simulink model "test"  (R2019b)
settings: Solver=VariableStepAuto  StartTime=0.0  StopTime=0.05  RelTol=1e-3
libraries: powerlib x11, simulink x3, dspsigops x1
settings Model: Creator=29721  LastModifiedBy=29721

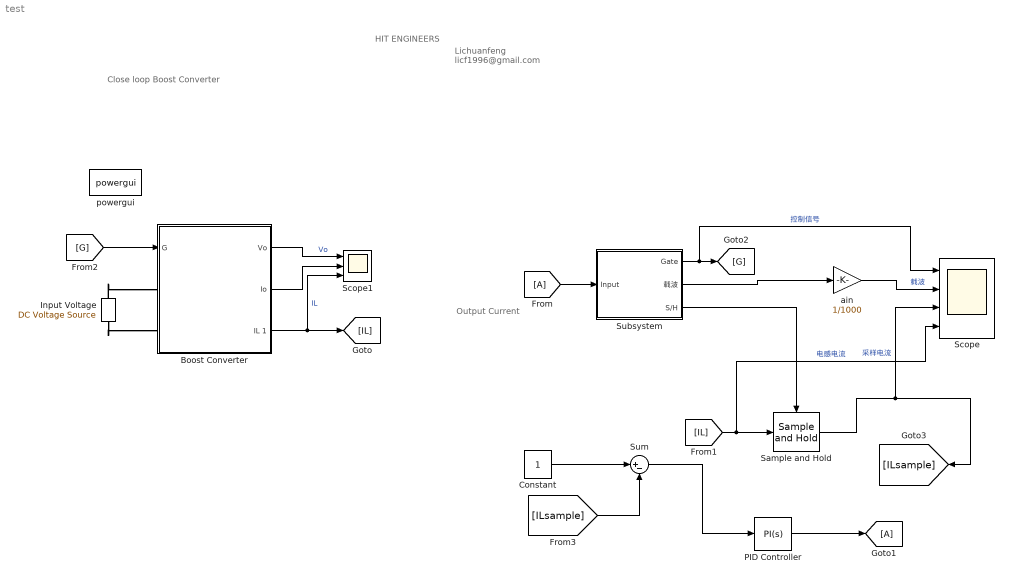
== system test ==
  note: HIT
      | ENGINEERS
  note: Lichuanfeng
      | licf1996@gmail.com
  note: Output Current
  note: Close loop Boost Converter
  Boost Converter : Subsystem  mask{R=20, L=5000e-6, C=220e-6}
      mask prompts: R "Resitor"; L "Inductor"; C "Capacitor"
  Constant : Constant
  Input Voltage : powerlib/Electrical Sources/DC Voltage Source  Amplitude=5  Measurements=None
  PID Controller : simulink/Continuous/PID Controller  Controller=PI  Form=Parallel  TimeDomain=Continuous-time  SampleTime=-1  IntegratorMethod=Forward Euler  FilterMethod=Forward Euler  ControllerParametersSource=internal  P=5000  I=20000  D=0  UseFilter=on  N=100  TunerSelectOption=Transfer Function Based (PID Tuner App)  InitialConditionSource=internal  InitialConditionForIntegrator=0  InitialConditionForFilter=0  DifferentiatorICPrevScaledInput=0  ExternalReset=none  TrackingMode=off  Kt=1  LimitOutput=off  UpperSaturationLimit=inf  LowerSaturationLimit=-inf  LinearizeAsGain=on  AntiWindupMode=none  Kb=1  POutMin=[]  POutMax=[]  IOutMin=[]  IOutMax=[]  DOutMin=[]  DOutMax=[]  NOutMin=[]  NOutMax=[]  SumOutMin=[]  SumOutMax=[]  SaturationOutMin=[]  SaturationOutMax=[]  PParamMin=[]  PParamMax=[]  IParamMin=[]  IParamMax=[]  DParamMin=[]  DParamMax=[]  NParamMin=[]  NParamMax=[]  KbParamMin=[]  KbParamMax=[]  KtParamMin=[]  KtParamMax=[]  KbOutMin=[]  KbOutMax=[]  KtOutMin=[]  KtOutMax=[]  IntegratorOutMin=[]  IntegratorOutMax=[]  FilterOutMin=[]  FilterOutMax=[]  SumI1OutMin=[]  SumI1OutMax=[]  SumI2OutMin=[]  SumI2OutMax=[]  SumI3OutMin=[]  SumI3OutMax=[]  SumI4OutMin=[]  SumI4OutMax=[]  SumDOutMin=[]  SumDOutMax=[]  DifferentiatorOutMin=[]  DifferentiatorOutMax=[]  FilterDiffOutCoefMin=[]  FilterDiffOutCoefMax=[]  ReciprocalOutMin=[]  ReciprocalOutMax=[]  SumDenOutMin=[]  SumDenOutMax=[]  SumNumOutMin=[]  SumNumOutMax=[]  DivideOutMin=[]  DivideOutMax=[]  IntegratorContinuousStateAttributes=''  IntegratorStateMustResolveToSignalObject=off  IntegratorRTWStateStorageClass=Auto  FilterContinuousStateAttributes=''  FilterStateMustResolveToSignalObject=off  FilterRTWStateStorageClass=Auto  ParallelPVariant=InternalParameters  IdealPVariant=Disabled  IVariant=InternalParameters  DVariant=Disabled  IntegratorVariant=Continuous  SatVariant=Disabled  AWVariant=Passthrough  PCopyVariant=Disabled  TRVariant=Disabled  FdbkBlocksVariant=Forward  IdealPFdbkVariant=Disabled  SatFdbkVariant=Disabled  DerivativeFilterVariant=Disabled  NVariant=Disabled  NCopyVariant=Disabled_SignalSpec  FilterICVariant=Disabled  IntegratorICVariant=InternalICs  ExternalResetVariant=Disabled  TRSumVariant=Passthrough  SumFdbkVariant=Disabled  SumVariant=Sum_PI
  Sample and Hold : dspsigops/Sample and Hold  trig=Rising edge  initCond=0  latchinput=off
  Scope : Scope  NumInputPorts=4
  Scope1 : Scope  NumInputPorts=3
  Subsystem : Subsystem  mask{Fs=100e3}
      mask prompts: Fs "swicthing frequency"
  Sum : Sum  Inputs=|+-
  ain : Gain  Gain=1/1000
  powergui : powerlib/powergui  Priority=1  SimulationMode=Discrete  SampleTime=1e-7  frequency=60  Iterations=50  frequencyindice=0  Pbase=100e6  ErrMax=1e-4  UnitsV=kV  UnitsW=MW  buscounter=0  FunctionMessages=off  echomessages=off  EnableUseOfTLC=off  CurrentSourceSwitches=off  DisableSnubberDevices=off  DisableRonSwitches=off  DisableVfSwitches=off  DisplayEquations=off  AutomaticDiscreteSolvers=off  SolverType=Tustin/Backward Euler (TBE)  Interpol=off  ExternalGateDelay=off  methode=off  Ts=100  x0status=blocks  SPID=on  SwTol=0  HookPort=off  NonlinearTolerance=1e-4  nMaxIteration=100  ContinueOnMaxIteration=off  RestoreLinks=warning  ResistiveCurrentMeasurement=off  Frange=[0:2:500]  Ylog=off  Xlog=on  ShowGrid=off  save=off  variable=ZData  structure=0  ZoomFFT=off  StartTime=0.0  cycles=1  DisplayStyle=1  fundamental=60  FreqAxis=off  MaxFrequency=1000  frequencyindicesteady=1  RmsSteady=1  display=off
  wires:
  Subsystem/2(载波) -> ain/1
  Subsystem/3(S/H) -> Sample and Hold/Trigger
  [IL] -> Scope/4, Sample and Hold/1  "电感电流"
  [A] -> Subsystem/1(Input)
  PID Controller/1 -> [A]
  Subsystem/1(Gate) -> Scope/1, [G]  "控制信号"
  Constant/1 -> Sum/1
  [ILsample] -> Sum/2
  Sum/1 -> PID Controller/1
  Boost Converter/1("Vo ") -> Scope1/1  "Vo"
  Boost Converter/2("Io ") -> Scope1/2
  [G] -> Boost Converter/1(G)
  Boost Converter/3(IL 1) -> Scope1/3, [IL]  "IL"
  Sample and Hold/1 -> Scope/3, [ILsample]  "采样电流"
  ain/1 -> Scope/2  "载波"
  connections:
  Input Voltage/LConn1 -- Boost Converter/LConn2
  Input Voltage/RConn1 -- Boost Converter/LConn1

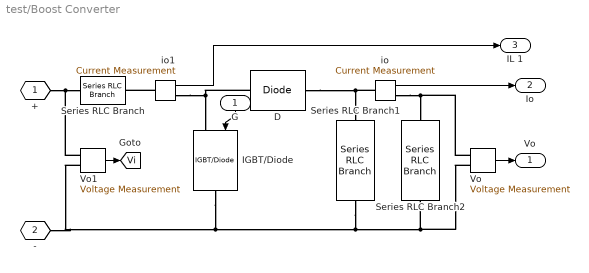
== system test/Boost Converter ==
  G : Inport
  D : powerlib/Power Electronics/Diode  Ron=0.001  Lon=0  Vf=0.001  IC=0  UseSnubber=off  Rs=500  Cs=250e-9  Measurements=off
  IGBT/Diode : powerlib/Power Electronics/IGBT//Diode  Ron=1e-3  Rs=1e5  Cs=inf  Measurements=off
  Series RLC Branch : powerlib/Elements/Series RLC Branch  LConnTagsString=__new0  RConnTagsString=__new0  BranchType=L  Resistance=1  Inductance=L  SetiL0=off  InitialCurrent=0  Capacitance=1e-6  Setx0=off  InitialVoltage=0  Measurements=None
  Series RLC Branch1 : powerlib/Elements/Series RLC Branch  LConnTagsString=__new0  RConnTagsString=__new0  BranchType=C  Resistance=1  Inductance=1e-3  SetiL0=off  InitialCurrent=0  Capacitance=C  Setx0=off  InitialVoltage=0  Measurements=None
  Series RLC Branch2 : powerlib/Elements/Series RLC Branch  LConnTagsString=__new0  RConnTagsString=__new0  BranchType=R  Resistance=R  Inductance=1e-3  SetiL0=off  InitialCurrent=0  Capacitance=220e-6  Setx0=off  InitialVoltage=0  Measurements=None
  Vo : powerlib/Measurements/Voltage Measurement  PhasorSimulation=off  OutputType=Complex  PSBequivalent=0
  Vo1 : powerlib/Measurements/Voltage Measurement  PhasorSimulation=off  OutputType=Complex  PSBequivalent=0
  io : powerlib/Measurements/Current Measurement  PhasorSimulation=off  OutputType=Complex  PSBequivalent=0
  io1 : powerlib/Measurements/Current Measurement  PhasorSimulation=off  OutputType=Complex  PSBequivalent=0
  + : PMIOPort  Tag=PMCPort  Side=Left
  - : PMIOPort  Tag=PMCPort  Port=2  Side=Left
  "Vo " : Outport
  "Io " : Outport  Port=2
  IL 1 : Outport  Port=3
  tag scope: Vi=global
  wires:
  Vo/1 -> "Vo "/1
  G/1 -> IGBT/Diode/1
  io/1 -> "Io "/1
  Vo1/1 -> [Vi]
  io1/1 -> IL 1/1
  connections:
  Vo/LConn1 -- io/RConn1 -- Series RLC Branch2/LConn1
  IGBT/Diode/RConn1 -- Vo1/LConn2 -- -/RConn1 -- Vo/LConn2 -- Series RLC Branch2/RConn1 -- Series RLC Branch1/RConn1
  D/LConn1 -- io1/RConn1 -- IGBT/Diode/LConn1
  Vo1/LConn1 -- +/RConn1 -- Series RLC Branch/LConn1
  D/RConn1 -- io/LConn1 -- Series RLC Branch1/LConn1
  io1/LConn1 -- Series RLC Branch/RConn1

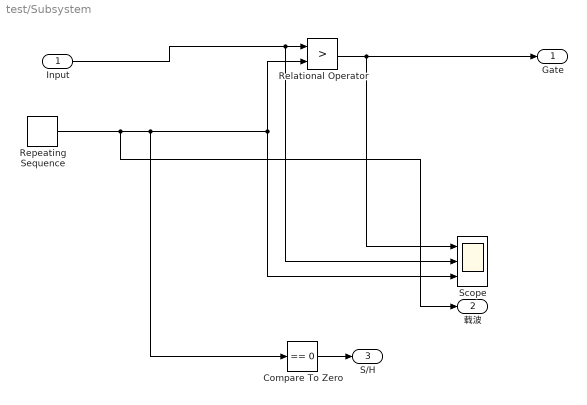
== system test/Subsystem ==
  Input : Inport
  Compare To Zero : simulink/Logic and Bit Operations/Compare To Zero  relop===  OutDataTypeStr=boolean
  Relational Operator : RelationalOperator  Operator=>  OutDataTypeStr=boolean  RndMeth=Simplest
  Repeating Sequence : simulink/Sources/Repeating Sequence  rep_seq_t=[0 1./Fs./2 1./Fs]  rep_seq_y=[0 1000 0]
  Scope : Scope  NumInputPorts=3
  Gate : Outport
  载波 : Outport  Port=2
  S/H : Outport  Port=3
  wires:
  Input/1 -> Scope/2, Relational Operator/1
  Compare To Zero/1 -> S/H/1
  Relational Operator/1 -> Scope/1, Gate/1
  Repeating Sequence/1 -> 载波/1, Compare To Zero/1, Relational Operator/2, Scope/3
